simulink model "NRC_Base_Rocket"  (R2025a)
settings: Solver=VariableStepAuto  StartTime=0.0  StopTime=10.0  RelTol=1e-3
settings Model: Creator=jakeo  LastModifiedBy=lukef

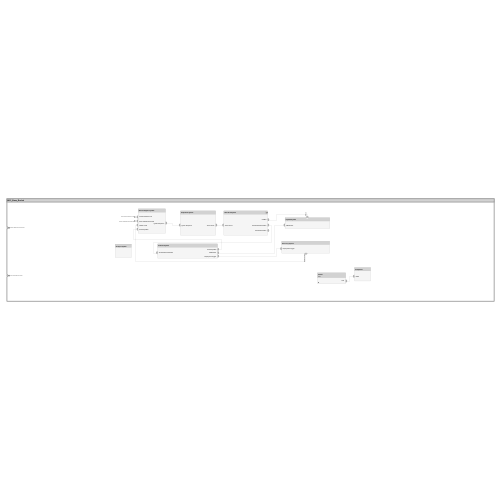
[thumbnail: Simulink's stored preview of the top-level diagram]
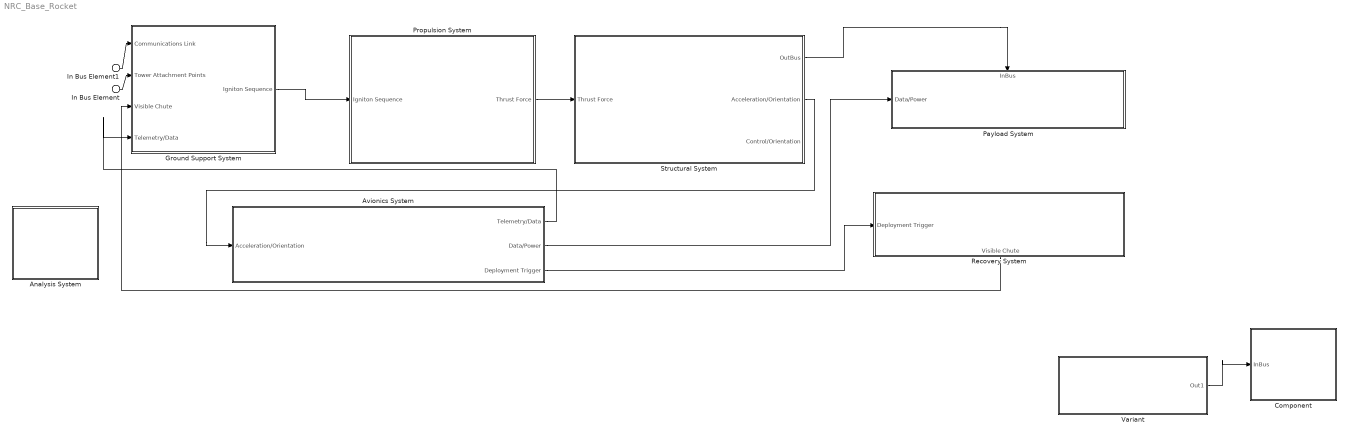
== system NRC_Base_Rocket ==
  In Bus Element : Inport  PortName=Tower Attachment Points
  In Bus Element1 : Inport  Port=2  PortName=Communications Link
  Analysis System : Subsystem
      settings: PortSchema="{\"entries\":[{\"content\":{\"headerSize\":26,\"margin\":15,\"minimumSpacing\":25,\"sides\":[{\"content\":{},\"type\":\"ConnectorPlacement.EquallySpacedRectSide\",\"uuid\":\"cc45333b-0876-4849-98d5-148de8a70f6b\"},{\"content\":{\"side\":\"RIGHT\"},\"type\":\"ConnectorPlacement.EquallySpacedRectSide\",\"uuid\":\"6d7662cc-0b93-4c22-b72a-22299e415e66\"},{\"content\":{\"side\":\"TOP\"},\"type\":\"ConnectorPlacement.EquallySpacedRectSide\",\"uuid\":\"98fed930-52bb-4e3d-bf56-50c036dee122\"}]},\"type\":\"ConnectorPlacement.EquallySpacedConnector\",\"uuid\":\"dfbe24ca-e965-4cbc-a32c-fe604c746b0d\"}],\"packageUris\":[\"http://schema.mathworks.com/mf0/Connector/R2020b\"],\"version\":\"1.0\"}"
  Avionics System : Subsystem
      settings: PortSchema="{\"entries\":[{\"content\":{\"headerSize\":26,\"margin\":15,\"minimumSpacing\":25,\"sides\":[{\"content\":{\"connectorIds\":[\"In1\"]},\"type\":\"ConnectorPlacement.EquallySpacedRectSide\",\"uuid\":\"6d56020f-32f3-4fce-baf0-a88f7155ace1\"},{\"content\":{\"connectorIds\":[\"Out1\",\"Out2\",\"Out3\"],\"side\":\"RIGHT\"},\"type\":\"ConnectorPlacement.EquallySpacedRectSide\",\"uuid\":\"c9981725-d77c-44c3-a293-bb000501b1f7\"},{\"content\":{\"side\":\"TOP\"},\"type\":\"ConnectorPlacement.EquallySpacedRectSide\",\"uuid\":\"9359d402-59c0-4829-a327-e8f675a7e108\"}]},\"type\":\"ConnectorPlacement.EquallySpacedConnector\",\"uuid\":\"22d4e63e-7f95-4c47-b029-dffe7490f4e3\"}],\"packageUris\":[\"http://schema.mathworks.com/mf0/Connector/R2020b\"],\"version\":\"1.0\"}"
  Component : Subsystem
      settings: PortSchema="{\"entries\":[{\"content\":{\"headerSize\":26,\"margin\":15,\"minimumSpacing\":25,\"sides\":[{\"content\":{\"connectorIds\":[\"In1\"]},\"type\":\"ConnectorPlacement.EquallySpacedRectSide\",\"uuid\":\"149126d5-b382-4b3b-94d2-e61d8a0b4f28\"},{\"content\":{\"side\":\"RIGHT\"},\"type\":\"ConnectorPlacement.EquallySpacedRectSide\",\"uuid\":\"9a27b6fc-3a4b-4444-8ae7-89bbe354237e\"},{\"content\":{\"side\":\"TOP\"},\"type\":\"ConnectorPlacement.EquallySpacedRectSide\",\"uuid\":\"ab34e53a-3e98-4f6d-b88d-ea909e518358\"}]},\"type\":\"ConnectorPlacement.EquallySpacedConnector\",\"uuid\":\"643790ba-b357-4d50-8632-6a2082f7e936\"}],\"packageUris\":[\"http://schema.mathworks.com/mf0/Connector/R2020b\"],\"version\":\"1.0\"}"
  Ground Support System : Subsystem
      settings: PortSchema="{\"entries\":[{\"content\":{\"headerSize\":26,\"margin\":15,\"minimumSpacing\":25,\"sides\":[{\"content\":{\"connectorIds\":[\"In1\",\"In4\",\"In3\",\"In2\"]},\"type\":\"ConnectorPlacement.EquallySpacedRectSide\",\"uuid\":\"6d56020f-32f3-4fce-baf0-a88f7155ace1\"},{\"content\":{\"connectorIds\":[\"Out1\"],\"side\":\"RIGHT\"},\"type\":\"ConnectorPlacement.EquallySpacedRectSide\",\"uuid\":\"c9981725-d77c-44c3-a293-bb000501b1f7\"},{\"content\":{\"side\":\"TOP\"},\"type\":\"ConnectorPlacement.EquallySpacedRectSide\",\"uuid\":\"9359d402-59c0-4829-a327-e8f675a7e108\"},{\"content\":{\"side\":\"BOTTOM\"},\"type\":\"ConnectorPlacement.EquallySpacedRectSide\",\"uuid\":\"0562d536-5ab7-4f95-b231-de77c5a317a2\"}]},\"type\":\"ConnectorPlacement.EquallySpacedConnector\",\"uuid\":\"22d4e63e-7f95-4c47-b029-dffe7490f4e3\"}],\"packageUris\":[\"http://schema.mathworks.com/mf0/Connector/R2020b\"],\"version\":\"1.0\"}"
  Payload System : Subsystem
      settings: PortSchema="{\"entries\":[{\"content\":{\"headerSize\":26,\"margin\":15,\"minimumSpacing\":25,\"sides\":[{\"content\":{\"connectorIds\":[\"In2\"]},\"type\":\"ConnectorPlacement.EquallySpacedRectSide\",\"uuid\":\"6d56020f-32f3-4fce-baf0-a88f7155ace1\"},{\"content\":{\"side\":\"RIGHT\"},\"type\":\"ConnectorPlacement.EquallySpacedRectSide\",\"uuid\":\"c9981725-d77c-44c3-a293-bb000501b1f7\"},{\"content\":{\"connectorIds\":[\"In1\"],\"side\":\"TOP\"},\"type\":\"ConnectorPlacement.EquallySpacedRectSide\",\"uuid\":\"9359d402-59c0-4829-a327-e8f675a7e108\"}]},\"type\":\"ConnectorPlacement.EquallySpacedConnector\",\"uuid\":\"22d4e63e-7f95-4c47-b029-dffe7490f4e3\"}],\"packageUris\":[\"http://schema.mathworks.com/mf0/Connector/R2020b\"],\"version\":\"1.0\"}"
  Propulsion System : Subsystem
      settings: PortSchema="{\"entries\":[{\"content\":{\"headerSize\":26,\"margin\":15,\"minimumSpacing\":25,\"sides\":[{\"content\":{\"connectorIds\":[\"In1\"]},\"type\":\"ConnectorPlacement.EquallySpacedRectSide\",\"uuid\":\"6d56020f-32f3-4fce-baf0-a88f7155ace1\"},{\"content\":{\"connectorIds\":[\"Out1\"],\"side\":\"RIGHT\"},\"type\":\"ConnectorPlacement.EquallySpacedRectSide\",\"uuid\":\"c9981725-d77c-44c3-a293-bb000501b1f7\"},{\"content\":{\"side\":\"TOP\"},\"type\":\"ConnectorPlacement.EquallySpacedRectSide\",\"uuid\":\"9359d402-59c0-4829-a327-e8f675a7e108\"},{\"content\":{\"side\":\"BOTTOM\"},\"type\":\"ConnectorPlacement.EquallySpacedRectSide\",\"uuid\":\"2f60ee6a-ee89-41bf-8f54-e5ad8be751a0\"}]},\"type\":\"ConnectorPlacement.EquallySpacedConnector\",\"uuid\":\"22d4e63e-7f95-4c47-b029-dffe7490f4e3\"}],\"packageUris\":[\"http://schema.mathworks.com/mf0/Connector/R2020b\"],\"version\":\"1.0\"}"
  Recovery System : Subsystem
      settings: PortSchema="{\"entries\":[{\"content\":{\"headerSize\":26,\"margin\":15,\"minimumSpacing\":25,\"sides\":[{\"content\":{\"connectorIds\":[\"In1\"]},\"type\":\"ConnectorPlacement.EquallySpacedRectSide\",\"uuid\":\"6d56020f-32f3-4fce-baf0-a88f7155ace1\"},{\"content\":{\"side\":\"RIGHT\"},\"type\":\"ConnectorPlacement.EquallySpacedRectSide\",\"uuid\":\"c9981725-d77c-44c3-a293-bb000501b1f7\"},{\"content\":{\"side\":\"TOP\"},\"type\":\"ConnectorPlacement.EquallySpacedRectSide\",\"uuid\":\"9359d402-59c0-4829-a327-e8f675a7e108\"},{\"content\":{\"connectorIds\":[\"Out1\"],\"side\":\"BOTTOM\"},\"type\":\"ConnectorPlacement.EquallySpacedRectSide\",\"uuid\":\"84cb8274-0faa-44eb-ac5a-c7f9ad04c935\"}]},\"type\":\"ConnectorPlacement.EquallySpacedConnector\",\"uuid\":\"22d4e63e-7f95-4c47-b029-dffe7490f4e3\"}],\"packageUris\":[\"http://schema.mathworks.com/mf0/Connector/R2020b\"],\"version\":\"1.0\"}"
  Structural System : Subsystem
      settings: PortSchema="{\"entries\":[{\"content\":{\"headerSize\":26,\"margin\":15,\"minimumSpacing\":25,\"sides\":[{\"content\":{\"connectorIds\":[\"In1\"]},\"type\":\"ConnectorPlacement.EquallySpacedRectSide\",\"uuid\":\"6d56020f-32f3-4fce-baf0-a88f7155ace1\"},{\"content\":{\"connectorIds\":[\"Out1\",\"Out2\",\"Out3\"],\"side\":\"RIGHT\"},\"type\":\"ConnectorPlacement.EquallySpacedRectSide\",\"uuid\":\"c9981725-d77c-44c3-a293-bb000501b1f7\"},{\"content\":{\"side\":\"TOP\"},\"type\":\"ConnectorPlacement.EquallySpacedRectSide\",\"uuid\":\"9359d402-59c0-4829-a327-e8f675a7e108\"}]},\"type\":\"ConnectorPlacement.EquallySpacedConnector\",\"uuid\":\"22d4e63e-7f95-4c47-b029-dffe7490f4e3\"}],\"packageUris\":[\"http://schema.mathworks.com/mf0/Connector/R2020b\"],\"version\":\"1.0\"}"
  Variant : Subsystem  Variant=on  VariantControlMode=label  LabelModeActiveChoice=true
      settings: PortSchema="{\"entries\":[{\"content\":{\"headerSize\":38,\"margin\":15,\"minimumSpacing\":25,\"sides\":[{\"content\":{},\"type\":\"ConnectorPlacement.EquallySpacedRectSide\",\"uuid\":\"22426e27-e721-4373-bd01-c2ce6c1da483\"},{\"content\":{\"connectorIds\":[\"Out1\"],\"side\":\"RIGHT\"},\"type\":\"ConnectorPlacement.EquallySpacedRectSide\",\"uuid\":\"3bf490f7-04b7-45dd-a121-e7c8eaa5110c\"},{\"content\":{\"side\":\"TOP\"},\"type\":\"ConnectorPlacement.EquallySpacedRectSide\",\"uuid\":\"9b0bb83b-2ca8-43f5-adcf-d733bff7ff31\"}]},\"type\":\"ConnectorPlacement.EquallySpacedConnector\",\"uuid\":\"56430b86-99d3-451e-8142-8b6f4eb799c1\"}],\"packageUris\":[\"http://schema.mathworks.com/mf0/Connector/R2020b\"],\"version\":\"1.0\"}"
  wires:
  In Bus Element/1 -> Ground Support System/4(Tower Attachment Points)
  Propulsion System/1(Thrust Force) -> Structural System/1(Thrust Force)
  Avionics System/3(Deployment Trigger) -> Recovery System/1(Deployment Trigger)
  Avionics System/2(Data/Power) -> Payload System/2(Data/Power)
  Avionics System/1(Telemetry/Data) -> Ground Support System/2(Telemetry/Data)
  Structural System/2(Acceleration/Orientation) -> Avionics System/1(Acceleration/Orientation)
  Ground Support System/1(Igniton Sequence) -> Propulsion System/1(Igniton Sequence)
  Structural System/1(OutBus) -> Payload System/1(InBus)
  Recovery System/1(Visible Chute) -> Ground Support System/3(Visible Chute)
  In Bus Element1/1 -> Ground Support System/1(Communications Link)
  Variant/1(Out1) -> Component/1(InBus)

== system NRC_Base_Rocket/Analysis System ==

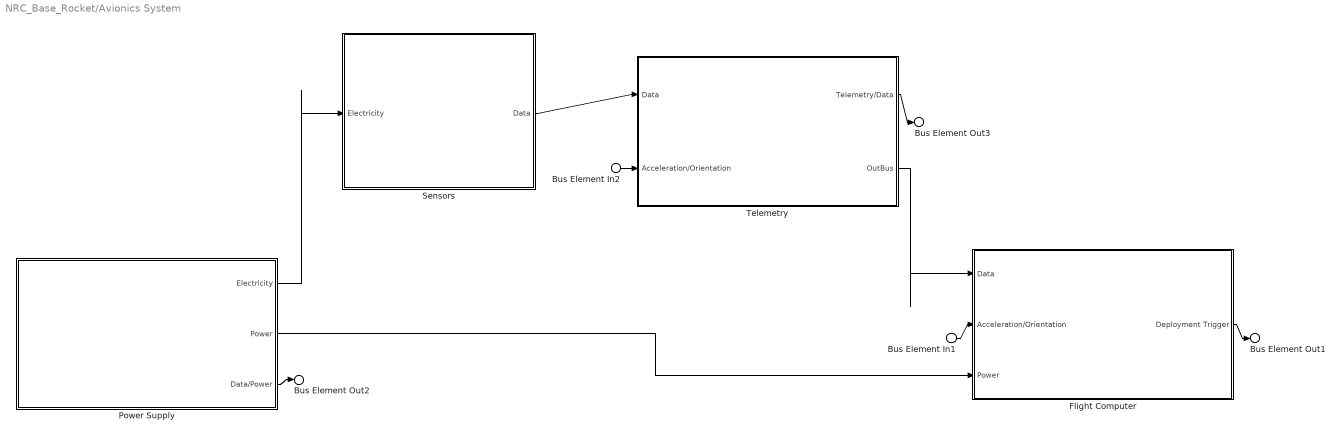
== system NRC_Base_Rocket/Avionics System ==
  Bus Element In1 : Inport  PortName=Acceleration/Orientation
  Bus Element In2 : Inport  PortName=Acceleration/Orientation
  Flight Computer : Subsystem
      settings: PortSchema="{\"entries\":[{\"content\":{\"headerSize\":26,\"margin\":15,\"minimumSpacing\":25,\"sides\":[{\"content\":{\"connectorIds\":[\"In1\",\"In2\",\"In3\"]},\"type\":\"ConnectorPlacement.EquallySpacedRectSide\",\"uuid\":\"6d56020f-32f3-4fce-baf0-a88f7155ace1\"},{\"content\":{\"connectorIds\":[\"Out1\"],\"side\":\"RIGHT\"},\"type\":\"ConnectorPlacement.EquallySpacedRectSide\",\"uuid\":\"c9981725-d77c-44c3-a293-bb000501b1f7\"},{\"content\":{\"side\":\"TOP\"},\"type\":\"ConnectorPlacement.EquallySpacedRectSide\",\"uuid\":\"9359d402-59c0-4829-a327-e8f675a7e108\"}]},\"type\":\"ConnectorPlacement.EquallySpacedConnector\",\"uuid\":\"22d4e63e-7f95-4c47-b029-dffe7490f4e3\"}],\"packageUris\":[\"http://schema.mathworks.com/mf0/Connector/R2020b\"],\"version\":\"1.0\"}"
  Power Supply : Subsystem
      settings: PortSchema="{\"entries\":[{\"content\":{\"headerSize\":26,\"margin\":15,\"minimumSpacing\":25,\"sides\":[{\"content\":{},\"type\":\"ConnectorPlacement.EquallySpacedRectSide\",\"uuid\":\"6d56020f-32f3-4fce-baf0-a88f7155ace1\"},{\"content\":{\"connectorIds\":[\"Out1\",\"Out2\",\"Out3\"],\"side\":\"RIGHT\"},\"type\":\"ConnectorPlacement.EquallySpacedRectSide\",\"uuid\":\"c9981725-d77c-44c3-a293-bb000501b1f7\"},{\"content\":{\"side\":\"TOP\"},\"type\":\"ConnectorPlacement.EquallySpacedRectSide\",\"uuid\":\"9359d402-59c0-4829-a327-e8f675a7e108\"}]},\"type\":\"ConnectorPlacement.EquallySpacedConnector\",\"uuid\":\"22d4e63e-7f95-4c47-b029-dffe7490f4e3\"}],\"packageUris\":[\"http://schema.mathworks.com/mf0/Connector/R2020b\"],\"version\":\"1.0\"}"
  Sensors : Subsystem
      settings: PortSchema="{\"entries\":[{\"content\":{\"headerSize\":26,\"margin\":15,\"minimumSpacing\":25,\"sides\":[{\"content\":{\"connectorIds\":[\"In1\"]},\"type\":\"ConnectorPlacement.EquallySpacedRectSide\",\"uuid\":\"6d56020f-32f3-4fce-baf0-a88f7155ace1\"},{\"content\":{\"connectorIds\":[\"Out1\"],\"side\":\"RIGHT\"},\"type\":\"ConnectorPlacement.EquallySpacedRectSide\",\"uuid\":\"c9981725-d77c-44c3-a293-bb000501b1f7\"},{\"content\":{\"side\":\"TOP\"},\"type\":\"ConnectorPlacement.EquallySpacedRectSide\",\"uuid\":\"9359d402-59c0-4829-a327-e8f675a7e108\"}]},\"type\":\"ConnectorPlacement.EquallySpacedConnector\",\"uuid\":\"22d4e63e-7f95-4c47-b029-dffe7490f4e3\"}],\"packageUris\":[\"http://schema.mathworks.com/mf0/Connector/R2020b\"],\"version\":\"1.0\"}"
  Telemetry : Subsystem
      settings: PortSchema="{\"entries\":[{\"content\":{\"headerSize\":26,\"margin\":15,\"minimumSpacing\":25,\"sides\":[{\"content\":{\"connectorIds\":[\"In1\",\"In2\"]},\"type\":\"ConnectorPlacement.EquallySpacedRectSide\",\"uuid\":\"6d56020f-32f3-4fce-baf0-a88f7155ace1\"},{\"content\":{\"connectorIds\":[\"Out1\",\"Out2\"],\"side\":\"RIGHT\"},\"type\":\"ConnectorPlacement.EquallySpacedRectSide\",\"uuid\":\"c9981725-d77c-44c3-a293-bb000501b1f7\"},{\"content\":{\"side\":\"TOP\"},\"type\":\"ConnectorPlacement.EquallySpacedRectSide\",\"uuid\":\"9359d402-59c0-4829-a327-e8f675a7e108\"}]},\"type\":\"ConnectorPlacement.EquallySpacedConnector\",\"uuid\":\"22d4e63e-7f95-4c47-b029-dffe7490f4e3\"}],\"packageUris\":[\"http://schema.mathworks.com/mf0/Connector/R2020b\"],\"version\":\"1.0\"}"
  Bus Element Out3 : Outport  PortName=Telemetry/Data
  Bus Element Out2 : Outport  Port=2  PortName=Data/Power
  Bus Element Out1 : Outport  Port=3  PortName=Deployment Trigger
  wires:
  Bus Element In1/1 -> Flight Computer/2(Acceleration/Orientation)
  Power Supply/2(Power) -> Flight Computer/3(Power)
  Power Supply/1(Electricity) -> Sensors/1(Electricity)
  Sensors/1(Data) -> Telemetry/1(Data)
  Telemetry/2(OutBus) -> Flight Computer/1(Data)
  Bus Element In2/1 -> Telemetry/2(Acceleration/Orientation)
  Telemetry/1(Telemetry/Data) -> Bus Element Out3/1
  Flight Computer/1(Deployment Trigger) -> Bus Element Out1/1
  Power Supply/3(Data/Power) -> Bus Element Out2/1

== system NRC_Base_Rocket/Component ==
  Bus Element In1 : Inport  PortName=InBus

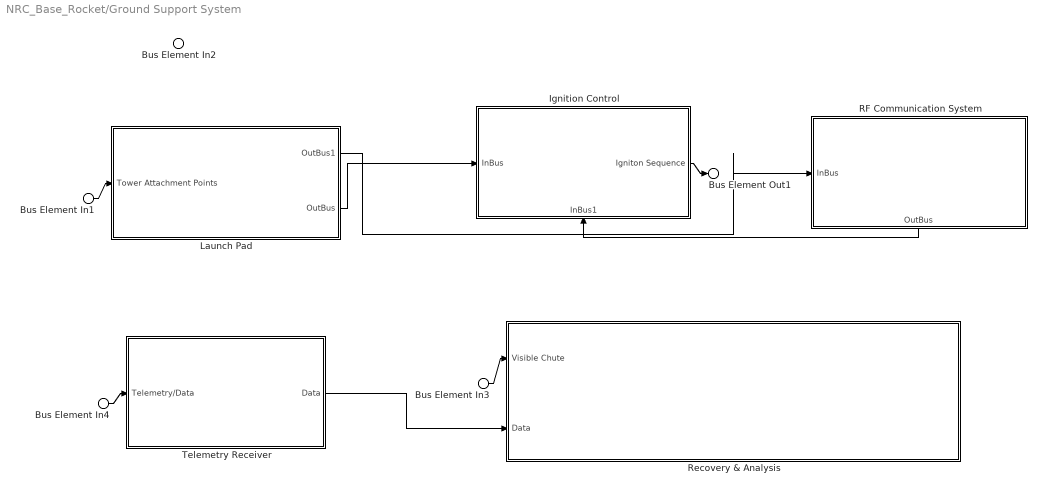
== system NRC_Base_Rocket/Ground Support System ==
  Bus Element In2 : Inport  PortName=Communications Link
  Bus Element In4 : Inport  Port=2  PortName=Telemetry/Data
  Bus Element In3 : Inport  Port=3  PortName=Visible Chute
  Bus Element In1 : Inport  Port=4  PortName=Tower Attachment Points
  Ignition Control : Subsystem
      settings: PortSchema="{\"entries\":[{\"content\":{\"headerSize\":26,\"margin\":15,\"minimumSpacing\":25,\"sides\":[{\"content\":{\"connectorIds\":[\"In2\"]},\"type\":\"ConnectorPlacement.EquallySpacedRectSide\",\"uuid\":\"6d56020f-32f3-4fce-baf0-a88f7155ace1\"},{\"content\":{\"connectorIds\":[\"Out1\"],\"side\":\"RIGHT\"},\"type\":\"ConnectorPlacement.EquallySpacedRectSide\",\"uuid\":\"c9981725-d77c-44c3-a293-bb000501b1f7\"},{\"content\":{\"side\":\"TOP\"},\"type\":\"ConnectorPlacement.EquallySpacedRectSide\",\"uuid\":\"9359d402-59c0-4829-a327-e8f675a7e108\"},{\"content\":{\"connectorIds\":[\"In1\"],\"side\":\"BOTTOM\"},\"type\":\"ConnectorPlacement.EquallySpacedRectSide\",\"uuid\":\"b26f05fe-132d-4676-8ad1-7fecac435fa8\"}]},\"type\":\"ConnectorPlacement.EquallySpacedConnector\",\"uuid\":\"22d4e63e-7f95-4c47-b029-dffe7490f4e3\"}],\"packageUris\":[\"http://schema.mathworks.com/mf0/Connector/R2020b\"],\"version\":\"1.0\"}"
  Launch Pad : Subsystem
      settings: PortSchema="{\"entries\":[{\"content\":{\"headerSize\":26,\"margin\":15,\"minimumSpacing\":25,\"sides\":[{\"content\":{\"connectorIds\":[\"In1\"]},\"type\":\"ConnectorPlacement.EquallySpacedRectSide\",\"uuid\":\"6d56020f-32f3-4fce-baf0-a88f7155ace1\"},{\"content\":{\"connectorIds\":[\"Out1\",\"Out2\"],\"side\":\"RIGHT\"},\"type\":\"ConnectorPlacement.EquallySpacedRectSide\",\"uuid\":\"c9981725-d77c-44c3-a293-bb000501b1f7\"},{\"content\":{\"side\":\"TOP\"},\"type\":\"ConnectorPlacement.EquallySpacedRectSide\",\"uuid\":\"9359d402-59c0-4829-a327-e8f675a7e108\"}]},\"type\":\"ConnectorPlacement.EquallySpacedConnector\",\"uuid\":\"22d4e63e-7f95-4c47-b029-dffe7490f4e3\"}],\"packageUris\":[\"http://schema.mathworks.com/mf0/Connector/R2020b\"],\"version\":\"1.0\"}"
  RF Communication System : Subsystem
      settings: PortSchema="{\"entries\":[{\"content\":{\"headerSize\":26,\"margin\":15,\"minimumSpacing\":25,\"sides\":[{\"content\":{\"connectorIds\":[\"In1\"]},\"type\":\"ConnectorPlacement.EquallySpacedRectSide\",\"uuid\":\"6d56020f-32f3-4fce-baf0-a88f7155ace1\"},{\"content\":{\"side\":\"RIGHT\"},\"type\":\"ConnectorPlacement.EquallySpacedRectSide\",\"uuid\":\"c9981725-d77c-44c3-a293-bb000501b1f7\"},{\"content\":{\"side\":\"TOP\"},\"type\":\"ConnectorPlacement.EquallySpacedRectSide\",\"uuid\":\"9359d402-59c0-4829-a327-e8f675a7e108\"},{\"content\":{\"connectorIds\":[\"Out1\"],\"side\":\"BOTTOM\"},\"type\":\"ConnectorPlacement.EquallySpacedRectSide\",\"uuid\":\"ccd2d326-55bc-4419-a15b-a3180bff0ee7\"}]},\"type\":\"ConnectorPlacement.EquallySpacedConnector\",\"uuid\":\"22d4e63e-7f95-4c47-b029-dffe7490f4e3\"}],\"packageUris\":[\"http://schema.mathworks.com/mf0/Connector/R2020b\"],\"version\":\"1.0\"}"
  Recovery & Analysis : Subsystem
      settings: PortSchema="{\"entries\":[{\"content\":{\"headerSize\":26,\"margin\":15,\"minimumSpacing\":25,\"sides\":[{\"content\":{\"connectorIds\":[\"In1\",\"In2\"]},\"type\":\"ConnectorPlacement.EquallySpacedRectSide\",\"uuid\":\"2e13f5a1-d12d-4e78-8c7d-b3419191e00e\"},{\"content\":{\"side\":\"RIGHT\"},\"type\":\"ConnectorPlacement.EquallySpacedRectSide\",\"uuid\":\"2e54f79d-d26c-4f1e-aad7-d167a8605581\"},{\"content\":{\"side\":\"TOP\"},\"type\":\"ConnectorPlacement.EquallySpacedRectSide\",\"uuid\":\"127632d1-acf1-4856-b80a-47a4730bf8fe\"}]},\"type\":\"ConnectorPlacement.EquallySpacedConnector\",\"uuid\":\"7fb5950c-eb56-4ad7-bb81-f4b7b8097c7f\"}],\"packageUris\":[\"http://schema.mathworks.com/mf0/Connector/R2020b\"],\"version\":\"1.0\"}"
  Telemetry Receiver : Subsystem
      settings: PortSchema="{\"entries\":[{\"content\":{\"headerSize\":26,\"margin\":15,\"minimumSpacing\":25,\"sides\":[{\"content\":{\"connectorIds\":[\"In1\"]},\"type\":\"ConnectorPlacement.EquallySpacedRectSide\",\"uuid\":\"6d56020f-32f3-4fce-baf0-a88f7155ace1\"},{\"content\":{\"connectorIds\":[\"Out1\"],\"side\":\"RIGHT\"},\"type\":\"ConnectorPlacement.EquallySpacedRectSide\",\"uuid\":\"c9981725-d77c-44c3-a293-bb000501b1f7\"},{\"content\":{\"side\":\"TOP\"},\"type\":\"ConnectorPlacement.EquallySpacedRectSide\",\"uuid\":\"9359d402-59c0-4829-a327-e8f675a7e108\"}]},\"type\":\"ConnectorPlacement.EquallySpacedConnector\",\"uuid\":\"22d4e63e-7f95-4c47-b029-dffe7490f4e3\"}],\"packageUris\":[\"http://schema.mathworks.com/mf0/Connector/R2020b\"],\"version\":\"1.0\"}"
  Bus Element Out1 : Outport  PortName=Igniton Sequence
  wires:
  Bus Element In3/1 -> Recovery & Analysis/1(Visible Chute)
  Bus Element In1/1 -> Launch Pad/1(Tower Attachment Points)
  Bus Element In4/1 -> Telemetry Receiver/1(Telemetry/Data)
  Telemetry Receiver/1(Data) -> Recovery & Analysis/2(Data)
  Launch Pad/2(OutBus) -> Ignition Control/2(InBus)
  Launch Pad/1(OutBus1) -> RF Communication System/1(InBus)
  RF Communication System/1(OutBus) -> Ignition Control/1(InBus1)
  Ignition Control/1(Igniton Sequence) -> Bus Element Out1/1

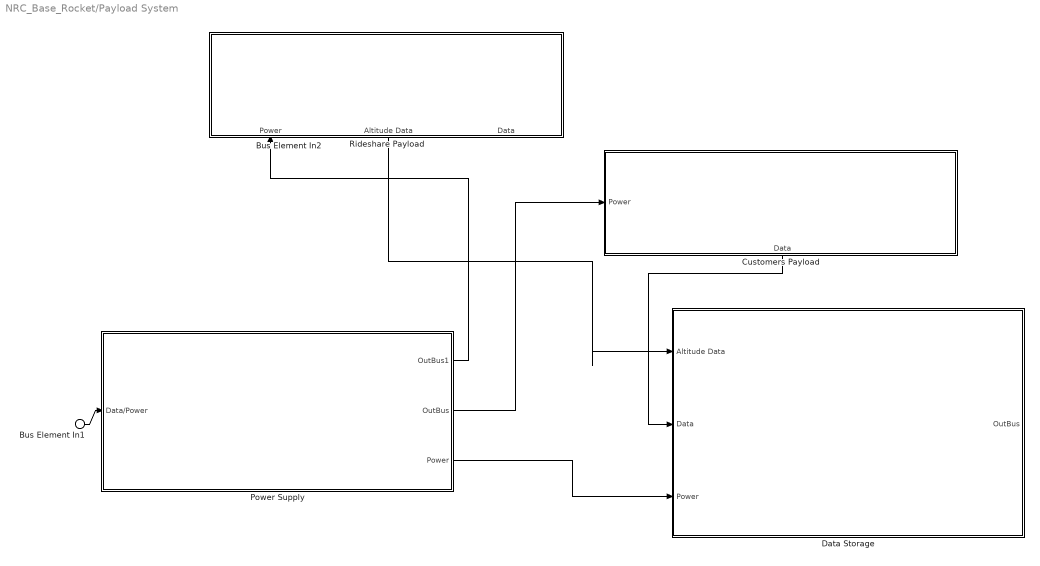
== system NRC_Base_Rocket/Payload System ==
  Bus Element In2 : Inport  PortName=InBus
  Bus Element In1 : Inport  Port=2  PortName=Data/Power
  Customers Payload : Subsystem
      settings: PortSchema="{\"entries\":[{\"content\":{\"headerSize\":26,\"margin\":15,\"minimumSpacing\":25,\"sides\":[{\"content\":{\"connectorIds\":[\"In1\"]},\"type\":\"ConnectorPlacement.EquallySpacedRectSide\",\"uuid\":\"6d56020f-32f3-4fce-baf0-a88f7155ace1\"},{\"content\":{\"side\":\"RIGHT\"},\"type\":\"ConnectorPlacement.EquallySpacedRectSide\",\"uuid\":\"c9981725-d77c-44c3-a293-bb000501b1f7\"},{\"content\":{\"side\":\"TOP\"},\"type\":\"ConnectorPlacement.EquallySpacedRectSide\",\"uuid\":\"9359d402-59c0-4829-a327-e8f675a7e108\"},{\"content\":{\"connectorIds\":[\"Out1\"],\"side\":\"BOTTOM\"},\"type\":\"ConnectorPlacement.EquallySpacedRectSide\",\"uuid\":\"17812ff1-462a-44f7-abf9-931c8845ebf9\"}]},\"type\":\"ConnectorPlacement.EquallySpacedConnector\",\"uuid\":\"22d4e63e-7f95-4c47-b029-dffe7490f4e3\"}],\"packageUris\":[\"http://schema.mathworks.com/mf0/Connector/R2020b\"],\"version\":\"1.0\"}"
  Data Storage : Subsystem
      settings: PortSchema="{\"entries\":[{\"content\":{\"headerSize\":26,\"margin\":15,\"minimumSpacing\":25,\"sides\":[{\"content\":{\"connectorIds\":[\"In1\",\"In2\",\"In3\"]},\"type\":\"ConnectorPlacement.EquallySpacedRectSide\",\"uuid\":\"6d56020f-32f3-4fce-baf0-a88f7155ace1\"},{\"content\":{\"connectorIds\":[\"Out1\"],\"side\":\"RIGHT\"},\"type\":\"ConnectorPlacement.EquallySpacedRectSide\",\"uuid\":\"c9981725-d77c-44c3-a293-bb000501b1f7\"},{\"content\":{\"side\":\"TOP\"},\"type\":\"ConnectorPlacement.EquallySpacedRectSide\",\"uuid\":\"9359d402-59c0-4829-a327-e8f675a7e108\"}]},\"type\":\"ConnectorPlacement.EquallySpacedConnector\",\"uuid\":\"22d4e63e-7f95-4c47-b029-dffe7490f4e3\"}],\"packageUris\":[\"http://schema.mathworks.com/mf0/Connector/R2020b\"],\"version\":\"1.0\"}"
  "Power Supply " : Subsystem
      settings: PortSchema="{\"entries\":[{\"content\":{\"headerSize\":26,\"margin\":15,\"minimumSpacing\":25,\"sides\":[{\"content\":{\"connectorIds\":[\"In1\"]},\"type\":\"ConnectorPlacement.EquallySpacedRectSide\",\"uuid\":\"6d56020f-32f3-4fce-baf0-a88f7155ace1\"},{\"content\":{\"connectorIds\":[\"Out1\",\"Out2\",\"Out3\"],\"side\":\"RIGHT\"},\"type\":\"ConnectorPlacement.EquallySpacedRectSide\",\"uuid\":\"c9981725-d77c-44c3-a293-bb000501b1f7\"},{\"content\":{\"side\":\"TOP\"},\"type\":\"ConnectorPlacement.EquallySpacedRectSide\",\"uuid\":\"9359d402-59c0-4829-a327-e8f675a7e108\"}]},\"type\":\"ConnectorPlacement.EquallySpacedConnector\",\"uuid\":\"22d4e63e-7f95-4c47-b029-dffe7490f4e3\"}],\"packageUris\":[\"http://schema.mathworks.com/mf0/Connector/R2020b\"],\"version\":\"1.0\"}"
  Rideshare Payload : Subsystem
      settings: PortSchema="{\"entries\":[{\"content\":{\"headerSize\":26,\"margin\":15,\"minimumSpacing\":25,\"sides\":[{\"content\":{},\"type\":\"ConnectorPlacement.EquallySpacedRectSide\",\"uuid\":\"2e13f5a1-d12d-4e78-8c7d-b3419191e00e\"},{\"content\":{\"side\":\"RIGHT\"},\"type\":\"ConnectorPlacement.EquallySpacedRectSide\",\"uuid\":\"2e54f79d-d26c-4f1e-aad7-d167a8605581\"},{\"content\":{\"side\":\"TOP\"},\"type\":\"ConnectorPlacement.EquallySpacedRectSide\",\"uuid\":\"127632d1-acf1-4856-b80a-47a4730bf8fe\"},{\"content\":{\"connectorIds\":[\"In1\",\"Out1\",\"Out2\"],\"side\":\"BOTTOM\"},\"type\":\"ConnectorPlacement.EquallySpacedRectSide\",\"uuid\":\"c99d9fe7-93a0-4b59-beae-ff6ce6a4fb80\"}]},\"type\":\"ConnectorPlacement.EquallySpacedConnector\",\"uuid\":\"7fb5950c-eb56-4ad7-bb81-f4b7b8097c7f\"}],\"packageUris\":[\"http://schema.mathworks.com/mf0/Connector/R2020b\"],\"version\":\"1.0\"}"
  wires:
  Bus Element In1/1 -> "Power Supply "/1(Data/Power)
  "Power Supply "/3(Power) -> Data Storage/3(Power)
  "Power Supply "/2(OutBus) -> Customers Payload/1(Power)
  Customers Payload/1(Data) -> Data Storage/2(Data)
  "Power Supply "/1(OutBus1) -> Rideshare Payload/1(Power)
  Rideshare Payload/1(Altitude Data) -> Data Storage/1(Altitude Data)

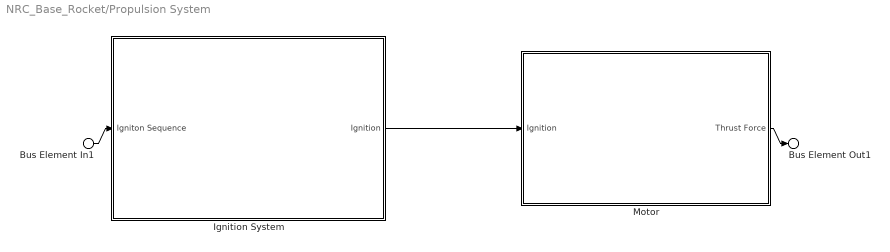
== system NRC_Base_Rocket/Propulsion System ==
  Bus Element In1 : Inport  PortName=Igniton Sequence
  Ignition System : Subsystem
      settings: PortSchema="{\"entries\":[{\"content\":{\"headerSize\":26,\"margin\":15,\"minimumSpacing\":25,\"sides\":[{\"content\":{\"connectorIds\":[\"In1\"]},\"type\":\"ConnectorPlacement.EquallySpacedRectSide\",\"uuid\":\"6d56020f-32f3-4fce-baf0-a88f7155ace1\"},{\"content\":{\"connectorIds\":[\"Out1\"],\"side\":\"RIGHT\"},\"type\":\"ConnectorPlacement.EquallySpacedRectSide\",\"uuid\":\"c9981725-d77c-44c3-a293-bb000501b1f7\"},{\"content\":{\"side\":\"TOP\"},\"type\":\"ConnectorPlacement.EquallySpacedRectSide\",\"uuid\":\"9359d402-59c0-4829-a327-e8f675a7e108\"}]},\"type\":\"ConnectorPlacement.EquallySpacedConnector\",\"uuid\":\"22d4e63e-7f95-4c47-b029-dffe7490f4e3\"}],\"packageUris\":[\"http://schema.mathworks.com/mf0/Connector/R2020b\"],\"version\":\"1.0\"}"
  "Motor " : Subsystem
      settings: PortSchema="{\"entries\":[{\"content\":{\"headerSize\":26,\"margin\":15,\"minimumSpacing\":25,\"sides\":[{\"content\":{\"connectorIds\":[\"In1\"]},\"type\":\"ConnectorPlacement.EquallySpacedRectSide\",\"uuid\":\"6d56020f-32f3-4fce-baf0-a88f7155ace1\"},{\"content\":{\"connectorIds\":[\"Out1\"],\"side\":\"RIGHT\"},\"type\":\"ConnectorPlacement.EquallySpacedRectSide\",\"uuid\":\"c9981725-d77c-44c3-a293-bb000501b1f7\"},{\"content\":{\"side\":\"TOP\"},\"type\":\"ConnectorPlacement.EquallySpacedRectSide\",\"uuid\":\"9359d402-59c0-4829-a327-e8f675a7e108\"}]},\"type\":\"ConnectorPlacement.EquallySpacedConnector\",\"uuid\":\"22d4e63e-7f95-4c47-b029-dffe7490f4e3\"}],\"packageUris\":[\"http://schema.mathworks.com/mf0/Connector/R2020b\"],\"version\":\"1.0\"}"
  Bus Element Out1 : Outport  PortName=Thrust Force
  wires:
  Bus Element In1/1 -> Ignition System/1(Igniton Sequence)
  Ignition System/1(Ignition) -> "Motor "/1(Ignition)
  "Motor "/1(Thrust Force) -> Bus Element Out1/1

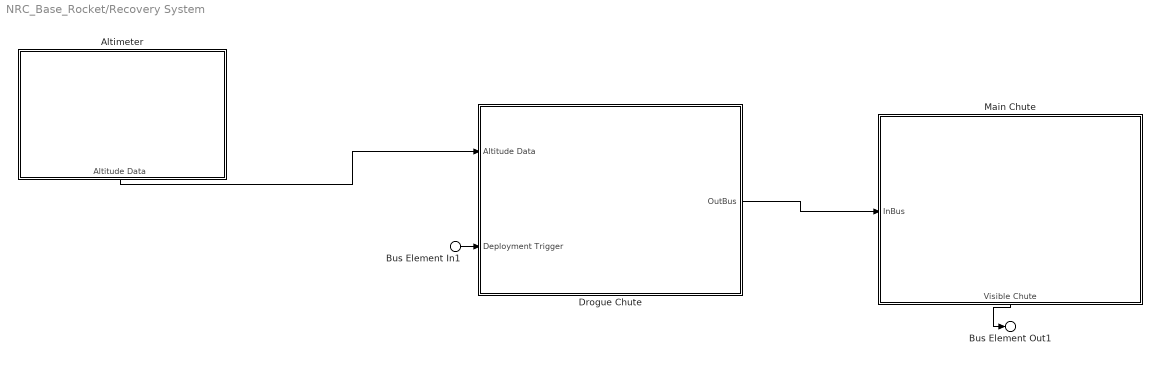
== system NRC_Base_Rocket/Recovery System ==
  Bus Element In1 : Inport  PortName=Deployment Trigger
  Altimeter : Subsystem
      settings: PortSchema="{\"entries\":[{\"content\":{\"headerSize\":26,\"margin\":15,\"minimumSpacing\":25,\"sides\":[{\"content\":{},\"type\":\"ConnectorPlacement.EquallySpacedRectSide\",\"uuid\":\"6d56020f-32f3-4fce-baf0-a88f7155ace1\"},{\"content\":{\"side\":\"RIGHT\"},\"type\":\"ConnectorPlacement.EquallySpacedRectSide\",\"uuid\":\"c9981725-d77c-44c3-a293-bb000501b1f7\"},{\"content\":{\"side\":\"TOP\"},\"type\":\"ConnectorPlacement.EquallySpacedRectSide\",\"uuid\":\"9359d402-59c0-4829-a327-e8f675a7e108\"},{\"content\":{\"connectorIds\":[\"Out1\"],\"side\":\"BOTTOM\"},\"type\":\"ConnectorPlacement.EquallySpacedRectSide\",\"uuid\":\"8243ea12-105d-44f7-b808-30ffb0a393f0\"}]},\"type\":\"ConnectorPlacement.EquallySpacedConnector\",\"uuid\":\"22d4e63e-7f95-4c47-b029-dffe7490f4e3\"}],\"packageUris\":[\"http://schema.mathworks.com/mf0/Connector/R2020b\"],\"version\":\"1.0\"}"
  Drogue Chute : Subsystem
      settings: PortSchema="{\"entries\":[{\"content\":{\"headerSize\":26,\"margin\":15,\"minimumSpacing\":25,\"sides\":[{\"content\":{\"connectorIds\":[\"In1\",\"In2\"]},\"type\":\"ConnectorPlacement.EquallySpacedRectSide\",\"uuid\":\"6d56020f-32f3-4fce-baf0-a88f7155ace1\"},{\"content\":{\"connectorIds\":[\"Out1\"],\"side\":\"RIGHT\"},\"type\":\"ConnectorPlacement.EquallySpacedRectSide\",\"uuid\":\"c9981725-d77c-44c3-a293-bb000501b1f7\"},{\"content\":{\"side\":\"TOP\"},\"type\":\"ConnectorPlacement.EquallySpacedRectSide\",\"uuid\":\"9359d402-59c0-4829-a327-e8f675a7e108\"}]},\"type\":\"ConnectorPlacement.EquallySpacedConnector\",\"uuid\":\"22d4e63e-7f95-4c47-b029-dffe7490f4e3\"}],\"packageUris\":[\"http://schema.mathworks.com/mf0/Connector/R2020b\"],\"version\":\"1.0\"}"
  Main Chute : Subsystem
      settings: PortSchema="{\"entries\":[{\"content\":{\"headerSize\":26,\"margin\":15,\"minimumSpacing\":25,\"sides\":[{\"content\":{\"connectorIds\":[\"In1\"]},\"type\":\"ConnectorPlacement.EquallySpacedRectSide\",\"uuid\":\"6d56020f-32f3-4fce-baf0-a88f7155ace1\"},{\"content\":{\"side\":\"RIGHT\"},\"type\":\"ConnectorPlacement.EquallySpacedRectSide\",\"uuid\":\"c9981725-d77c-44c3-a293-bb000501b1f7\"},{\"content\":{\"side\":\"TOP\"},\"type\":\"ConnectorPlacement.EquallySpacedRectSide\",\"uuid\":\"9359d402-59c0-4829-a327-e8f675a7e108\"},{\"content\":{\"connectorIds\":[\"Out1\"],\"side\":\"BOTTOM\"},\"type\":\"ConnectorPlacement.EquallySpacedRectSide\",\"uuid\":\"f809839c-bd2a-4c61-a037-fd3459666388\"}]},\"type\":\"ConnectorPlacement.EquallySpacedConnector\",\"uuid\":\"22d4e63e-7f95-4c47-b029-dffe7490f4e3\"}],\"packageUris\":[\"http://schema.mathworks.com/mf0/Connector/R2020b\"],\"version\":\"1.0\"}"
  Bus Element Out1 : Outport  PortName=Visible Chute
  wires:
  Bus Element In1/1 -> Drogue Chute/2(Deployment Trigger)
  Altimeter/1(Altitude Data) -> Drogue Chute/1(Altitude Data)
  Drogue Chute/1(OutBus) -> Main Chute/1(InBus)
  Main Chute/1(Visible Chute) -> Bus Element Out1/1

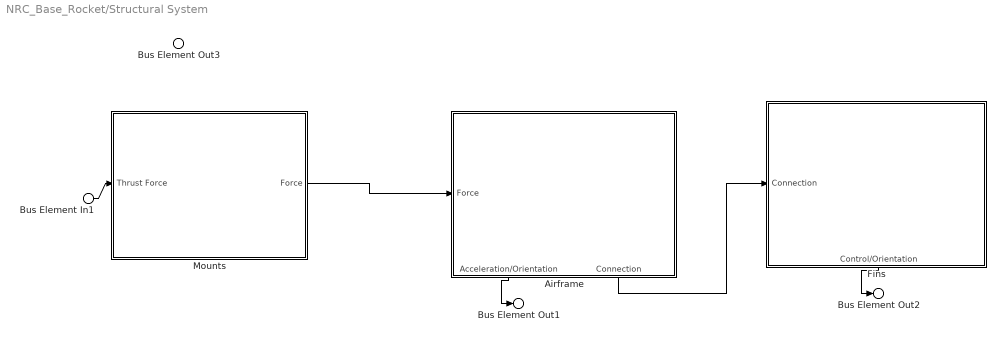
== system NRC_Base_Rocket/Structural System ==
  Bus Element In1 : Inport  PortName=Thrust Force
  Airframe : Subsystem
      settings: PortSchema="{\"entries\":[{\"content\":{\"headerSize\":26,\"margin\":15,\"minimumSpacing\":25,\"sides\":[{\"content\":{\"connectorIds\":[\"In1\"]},\"type\":\"ConnectorPlacement.EquallySpacedRectSide\",\"uuid\":\"6d56020f-32f3-4fce-baf0-a88f7155ace1\"},{\"content\":{\"side\":\"RIGHT\"},\"type\":\"ConnectorPlacement.EquallySpacedRectSide\",\"uuid\":\"c9981725-d77c-44c3-a293-bb000501b1f7\"},{\"content\":{\"side\":\"TOP\"},\"type\":\"ConnectorPlacement.EquallySpacedRectSide\",\"uuid\":\"9359d402-59c0-4829-a327-e8f675a7e108\"},{\"content\":{\"connectorIds\":[\"Out1\",\"Out2\"],\"side\":\"BOTTOM\"},\"type\":\"ConnectorPlacement.EquallySpacedRectSide\",\"uuid\":\"1e7e0694-c431-49bf-9519-4fa148c41ab4\"}]},\"type\":\"ConnectorPlacement.EquallySpacedConnector\",\"uuid\":\"22d4e63e-7f95-4c47-b029-dffe7490f4e3\"}],\"packageUris\":[\"http://schema.mathworks.com/mf0/Connector/R2020b\"],\"version\":\"1.0\"}"
  Fins : Subsystem
      settings: PortSchema="{\"entries\":[{\"content\":{\"headerSize\":26,\"margin\":15,\"minimumSpacing\":25,\"sides\":[{\"content\":{\"connectorIds\":[\"In1\"]},\"type\":\"ConnectorPlacement.EquallySpacedRectSide\",\"uuid\":\"6d56020f-32f3-4fce-baf0-a88f7155ace1\"},{\"content\":{\"side\":\"RIGHT\"},\"type\":\"ConnectorPlacement.EquallySpacedRectSide\",\"uuid\":\"c9981725-d77c-44c3-a293-bb000501b1f7\"},{\"content\":{\"side\":\"TOP\"},\"type\":\"ConnectorPlacement.EquallySpacedRectSide\",\"uuid\":\"9359d402-59c0-4829-a327-e8f675a7e108\"},{\"content\":{\"connectorIds\":[\"Out1\"],\"side\":\"BOTTOM\"},\"type\":\"ConnectorPlacement.EquallySpacedRectSide\",\"uuid\":\"934d0f44-d9ca-45cf-ac41-f0da4384728e\"}]},\"type\":\"ConnectorPlacement.EquallySpacedConnector\",\"uuid\":\"22d4e63e-7f95-4c47-b029-dffe7490f4e3\"}],\"packageUris\":[\"http://schema.mathworks.com/mf0/Connector/R2020b\"],\"version\":\"1.0\"}"
  Mounts : Subsystem
      settings: PortSchema="{\"entries\":[{\"content\":{\"headerSize\":26,\"margin\":15,\"minimumSpacing\":25,\"sides\":[{\"content\":{\"connectorIds\":[\"In1\"]},\"type\":\"ConnectorPlacement.EquallySpacedRectSide\",\"uuid\":\"6d56020f-32f3-4fce-baf0-a88f7155ace1\"},{\"content\":{\"connectorIds\":[\"Out1\"],\"side\":\"RIGHT\"},\"type\":\"ConnectorPlacement.EquallySpacedRectSide\",\"uuid\":\"c9981725-d77c-44c3-a293-bb000501b1f7\"},{\"content\":{\"side\":\"TOP\"},\"type\":\"ConnectorPlacement.EquallySpacedRectSide\",\"uuid\":\"9359d402-59c0-4829-a327-e8f675a7e108\"}]},\"type\":\"ConnectorPlacement.EquallySpacedConnector\",\"uuid\":\"22d4e63e-7f95-4c47-b029-dffe7490f4e3\"}],\"packageUris\":[\"http://schema.mathworks.com/mf0/Connector/R2020b\"],\"version\":\"1.0\"}"
  Bus Element Out3 : Outport  PortName=OutBus
  Bus Element Out1 : Outport  Port=2  PortName=Acceleration/Orientation
  Bus Element Out2 : Outport  Port=3  PortName=Control/Orientation
  wires:
  Bus Element In1/1 -> Mounts/1(Thrust Force)
  Mounts/1(Force) -> Airframe/1(Force)
  Airframe/2(Connection) -> Fins/1(Connection)
  Airframe/1(Acceleration/Orientation) -> Bus Element Out1/1
  Fins/1(Control/Orientation) -> Bus Element Out2/1

== system NRC_Base_Rocket/Variant ==
  Component : Subsystem  VariantControl=true
      settings: PortSchema="{\"entries\":[{\"content\":{\"headerSize\":26,\"margin\":15,\"minimumSpacing\":25,\"sides\":[{\"content\":{},\"type\":\"ConnectorPlacement.EquallySpacedRectSide\",\"uuid\":\"3697869b-a29e-41f0-b975-c76e09db82ee\"},{\"content\":{\"side\":\"RIGHT\"},\"type\":\"ConnectorPlacement.EquallySpacedRectSide\",\"uuid\":\"3b243a3d-994c-44c2-a8ac-06b646a41414\"},{\"content\":{\"side\":\"TOP\"},\"type\":\"ConnectorPlacement.EquallySpacedRectSide\",\"uuid\":\"a458fff4-a09e-47f2-acd2-6608413a4c15\"}]},\"type\":\"ConnectorPlacement.EquallySpacedConnector\",\"uuid\":\"d7f1f017-78a4-4f30-bf27-11b76259d801\"}],\"packageUris\":[\"http://schema.mathworks.com/mf0/Connector/R2020b\"],\"version\":\"1.0\"}"
  Component1 : Subsystem  VariantControl=false
      settings: PortSchema="{\"entries\":[{\"content\":{\"headerSize\":26,\"margin\":15,\"minimumSpacing\":25,\"sides\":[{\"content\":{},\"type\":\"ConnectorPlacement.EquallySpacedRectSide\",\"uuid\":\"3697869b-a29e-41f0-b975-c76e09db82ee\"},{\"content\":{\"side\":\"RIGHT\"},\"type\":\"ConnectorPlacement.EquallySpacedRectSide\",\"uuid\":\"3b243a3d-994c-44c2-a8ac-06b646a41414\"},{\"content\":{\"side\":\"TOP\"},\"type\":\"ConnectorPlacement.EquallySpacedRectSide\",\"uuid\":\"a458fff4-a09e-47f2-acd2-6608413a4c15\"}]},\"type\":\"ConnectorPlacement.EquallySpacedConnector\",\"uuid\":\"d7f1f017-78a4-4f30-bf27-11b76259d801\"}],\"packageUris\":[\"http://schema.mathworks.com/mf0/Connector/R2020b\"],\"version\":\"1.0\"}"
  Out1 : Outport

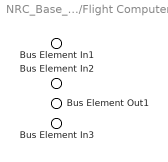
== system NRC_Base_Rocket/Avionics System/Flight Computer ==
  Bus Element In1 : Inport  PortName=Data
  Bus Element In2 : Inport  Port=2  PortName=Acceleration/Orientation
  Bus Element In3 : Inport  Port=3  PortName=Power
  Bus Element Out1 : Outport  PortName=Deployment Trigger

== system NRC_Base_Rocket/Avionics System/Power Supply ==
  Bus Element Out2 : Outport  PortName=Electricity
  Bus Element Out1 : Outport  Port=2  PortName=Power
  Bus Element Out3 : Outport  Port=3  PortName=Data/Power

== system NRC_Base_Rocket/Avionics System/Sensors ==
  Bus Element In1 : Inport  PortName=Electricity
  Bus Element Out1 : Outport  PortName=Data

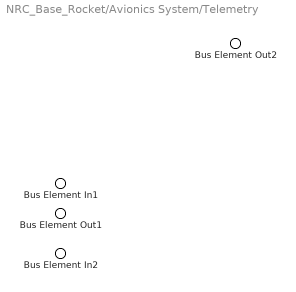
== system NRC_Base_Rocket/Avionics System/Telemetry ==
  Bus Element In1 : Inport  PortName=Data
  Bus Element In2 : Inport  Port=2  PortName=Acceleration/Orientation
  Bus Element Out2 : Outport  PortName=Telemetry/Data
  Bus Element Out1 : Outport  Port=2  PortName=OutBus

== system NRC_Base_Rocket/Ground Support System/Ignition Control ==
  Bus Element In2 : Inport  PortName=InBus1
  Bus Element In1 : Inport  Port=2  PortName=InBus
  Bus Element Out1 : Outport  PortName=Igniton Sequence

== system NRC_Base_Rocket/Ground Support System/Launch Pad ==
  Bus Element In1 : Inport  PortName=Tower Attachment Points
  Bus Element Out2 : Outport  PortName=OutBus1
  Bus Element Out1 : Outport  Port=2  PortName=OutBus

== system NRC_Base_Rocket/Ground Support System/RF Communication System ==
  Bus Element In1 : Inport  PortName=InBus
  Bus Element Out1 : Outport  PortName=OutBus

== system NRC_Base_Rocket/Ground Support System/Recovery & Analysis ==
  Bus Element In2 : Inport  PortName=Visible Chute
  Bus Element In1 : Inport  Port=2  PortName=Data

== system NRC_Base_Rocket/Ground Support System/Telemetry Receiver ==
  Bus Element In1 : Inport  PortName=Telemetry/Data
  Bus Element Out1 : Outport  PortName=Data

== system NRC_Base_Rocket/Payload System/Customers Payload ==
  Bus Element In1 : Inport  PortName=Power
  Bus Element Out1 : Outport  PortName=Data

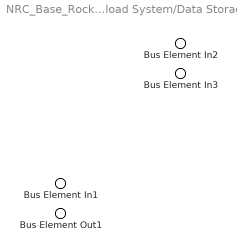
== system NRC_Base_Rocket/Payload System/Data Storage ==
  Bus Element In3 : Inport  PortName=Altitude Data
  Bus Element In2 : Inport  Port=2  PortName=Data
  Bus Element In1 : Inport  Port=3  PortName=Power
  Bus Element Out1 : Outport  PortName=OutBus

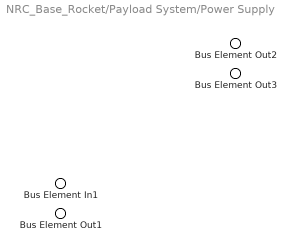
== system NRC_Base_Rocket/Payload System/Power Supply  ==
  Bus Element In1 : Inport  PortName=Data/Power
  Bus Element Out3 : Outport  PortName=OutBus1
  Bus Element Out2 : Outport  Port=2  PortName=OutBus
  Bus Element Out1 : Outport  Port=3  PortName=Power

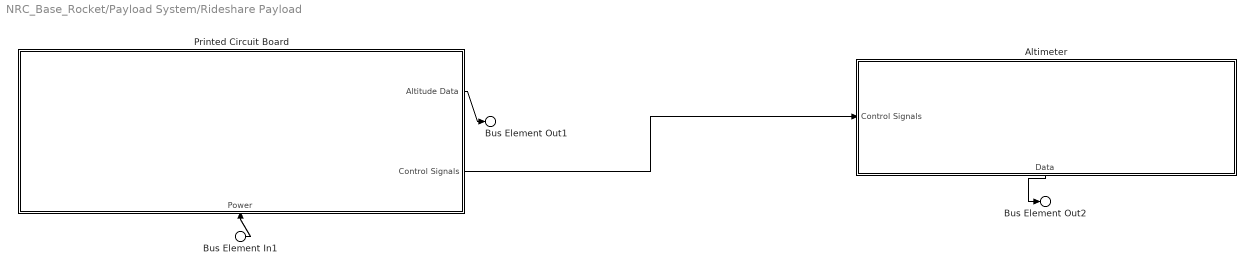
== system NRC_Base_Rocket/Payload System/Rideshare Payload ==
  Bus Element In1 : Inport  PortName=Power
  Altimeter : Subsystem
      settings: PortSchema="{\"entries\":[{\"content\":{\"headerSize\":26,\"margin\":15,\"minimumSpacing\":25,\"sides\":[{\"content\":{\"connectorIds\":[\"In1\"]},\"type\":\"ConnectorPlacement.EquallySpacedRectSide\",\"uuid\":\"2e13f5a1-d12d-4e78-8c7d-b3419191e00e\"},{\"content\":{\"side\":\"RIGHT\"},\"type\":\"ConnectorPlacement.EquallySpacedRectSide\",\"uuid\":\"2e54f79d-d26c-4f1e-aad7-d167a8605581\"},{\"content\":{\"side\":\"TOP\"},\"type\":\"ConnectorPlacement.EquallySpacedRectSide\",\"uuid\":\"127632d1-acf1-4856-b80a-47a4730bf8fe\"},{\"content\":{\"connectorIds\":[\"Out1\"],\"side\":\"BOTTOM\"},\"type\":\"ConnectorPlacement.EquallySpacedRectSide\",\"uuid\":\"4fc0a07c-a833-4ca9-b6fd-5fc8d4c0b5dc\"}]},\"type\":\"ConnectorPlacement.EquallySpacedConnector\",\"uuid\":\"7fb5950c-eb56-4ad7-bb81-f4b7b8097c7f\"}],\"packageUris\":[\"http://schema.mathworks.com/mf0/Connector/R2020b\"],\"version\":\"1.0\"}"
  Printed Circuit Board : Subsystem
      settings: PortSchema="{\"entries\":[{\"content\":{\"headerSize\":26,\"margin\":15,\"minimumSpacing\":25,\"sides\":[{\"content\":{},\"type\":\"ConnectorPlacement.EquallySpacedRectSide\",\"uuid\":\"2e13f5a1-d12d-4e78-8c7d-b3419191e00e\"},{\"content\":{\"connectorIds\":[\"Out1\",\"Out2\"],\"side\":\"RIGHT\"},\"type\":\"ConnectorPlacement.EquallySpacedRectSide\",\"uuid\":\"2e54f79d-d26c-4f1e-aad7-d167a8605581\"},{\"content\":{\"side\":\"TOP\"},\"type\":\"ConnectorPlacement.EquallySpacedRectSide\",\"uuid\":\"127632d1-acf1-4856-b80a-47a4730bf8fe\"},{\"content\":{\"connectorIds\":[\"In1\"],\"side\":\"BOTTOM\"},\"type\":\"ConnectorPlacement.EquallySpacedRectSide\",\"uuid\":\"84609f25-f9e8-4f57-ac2d-b4cbc4264e2d\"}]},\"type\":\"ConnectorPlacement.EquallySpacedConnector\",\"uuid\":\"7fb5950c-eb56-4ad7-bb81-f4b7b8097c7f\"}],\"packageUris\":[\"http://schema.mathworks.com/mf0/Connector/R2020b\"],\"version\":\"1.0\"}"
  Bus Element Out1 : Outport  PortName=Altitude Data
  Bus Element Out2 : Outport  Port=2  PortName=Data
  wires:
  Bus Element In1/1 -> Printed Circuit Board/1(Power)
  Printed Circuit Board/1(Altitude Data) -> Bus Element Out1/1
  Printed Circuit Board/2(Control Signals) -> Altimeter/1(Control Signals)
  Altimeter/1(Data) -> Bus Element Out2/1

== system NRC_Base_Rocket/Propulsion System/Ignition System ==
  Bus Element In1 : Inport  PortName=Igniton Sequence
  Bus Element Out1 : Outport  PortName=Ignition

== system NRC_Base_Rocket/Propulsion System/Motor  ==
  Bus Element In1 : Inport  PortName=Ignition
  Bus Element Out1 : Outport  PortName=Thrust Force

== system NRC_Base_Rocket/Recovery System/Altimeter ==
  Bus Element Out1 : Outport  PortName=Altitude Data

== system NRC_Base_Rocket/Recovery System/Drogue Chute ==
  Bus Element In2 : Inport  PortName=Altitude Data
  Bus Element In1 : Inport  Port=2  PortName=Deployment Trigger
  Bus Element Out1 : Outport  PortName=OutBus

== system NRC_Base_Rocket/Recovery System/Main Chute ==
  Bus Element In1 : Inport  PortName=InBus
  Bus Element Out1 : Outport  PortName=Visible Chute

== system NRC_Base_Rocket/Structural System/Airframe ==
  Bus Element In1 : Inport  PortName=Force
  Bus Element Out2 : Outport  PortName=Acceleration/Orientation
  Bus Element Out1 : Outport  Port=2  PortName=Connection

== system NRC_Base_Rocket/Structural System/Fins ==
  Bus Element In1 : Inport  PortName=Connection
  Bus Element Out1 : Outport  PortName=Control/Orientation

== system NRC_Base_Rocket/Structural System/Mounts ==
  Bus Element In1 : Inport  PortName=Thrust Force
  Bus Element Out1 : Outport  PortName=Force

== system NRC_Base_Rocket/Variant/Component ==

== system NRC_Base_Rocket/Variant/Component1 ==

== system NRC_Base_Rocket/Payload System/Rideshare Payload/Altimeter ==
  Bus Element In1 : Inport  PortName=Control Signals
  Bus Element Out1 : Outport  PortName=Data

== system NRC_Base_Rocket/Payload System/Rideshare Payload/Printed Circuit Board ==
  Bus Element In1 : Inport  PortName=Power
  Bus Element Out1 : Outport  PortName=Altitude Data
  Bus Element Out2 : Outport  Port=2  PortName=Control Signals
